simulink model "flightControlSystemV2"  (R2023a)
settings: Solver=ode3  StartTime=0  StopTime=TFinal  FixedStep=Ts  RelTol=1e-3  EnableMultiTasking=on
undefined symbols (not defined in the file or in its folder): codertarget, Controller, DiscIntNeverNeededParam, Discrete, Estimator, g, gray, init, orient_ref, pos_ref, Sensors, Time, Ts, var_acc_angle_N, var_bias_gyr_N, var_gyro_p_N, Vehicle
libraries: simulink x37, slpidlib x4, ctrlSharedLib x4, sharedtransform x3, parrotlib x1
(part 3 of 3)

== matlab function flightControlSystemV2/Image Processing System/MATLAB Function2 ==
  data: BW input; R input; G input; B input; state input; lineSteps input; len_center output; turn_angle output; state output; lineSteps output; R_out output; G_out output; B_out output; turn_angle input; turn input; turn output; correction output; angle input; angle output
function [len_center, turn_angle, state, lineSteps, R_out, G_out, B_out, turn, correction, angle] = droneGuidanceLines(BW, R, G, B, state, lineSteps, turn_angle, turn, angle)
    % Get image dimensions
    [rows, cols] = size(BW);

    turn_detected = false;
    turn_direction = 0;
    end_point_1 = [0,0];
    end_point_2 = [0,0];
    pinkColor = [255, 105, 180]; % RGB values for pink color
    greenColor = [0, 255, 0]; % RGB values for green color
    correction_thresh = 0.9;
    correction = 0;




    if state == 5
        turn = 0;
        state = 1;
    end
    
    % Define the drone's position (center of the image)
    drone_position = [round(rows/2), round(cols/2)];
    

    % Lengths of lines initialized to 0
    len_center = 0;
    len_left = 0;
    len_right = 0;
    len_left_or = 0;
    len_right_or = 0;
    len_back_left = 0;
    len_back_right = 0;
    len_left_corr = 0;
    len_right_corr = 0;
    
     % Step sizes for each line based on lineSteps array
    step_center = lineSteps(1,:);
    step_left = lineSteps(2,:);
    step_right = lineSteps(3,:);
    step_left_or = lineSteps(4,:);
    step_right_or = lineSteps(5,:);
    step_back_left = lineSteps(6,:);
    step_back_right = lineSteps(7,:);
    step_left_corr = [-step_center(2), step_center(1)]; 
    step_right_corr = [step_center(2), -step_center(1)]; 


    
    % Flags to check if lines should continue
    continue_center = true;
    continue_left = true;
    continue_right = true;
    continue_left_or = true;
    continue_right_or = true;
    continue_back_left = true;
    continue_back_right = true;
    continue_left_corr = true;
    continue_right_corr = true;



    % Initialize RGB values and lengths
    [len_center, R, G, B] = traceLine(drone_position, step_center, BW, R, G, B, pinkColor);
    [len_left, R, G, B] = traceLine(drone_position, step_left, BW, R, G, B, greenColor);
    [len_right, R, G, B] = traceLine(drone_position, step_right, BW, R, G, B, greenColor);
    [len_left_or, R, G, B] = traceLine(drone_position, step_left_or, BW, R, G, B, greenColor);
    [len_right_or, R, G, B] = traceLine(drone_position, step_right_or, BW, R, G, B, greenColor);
    [len_back_left, R, G, B] = traceLine(drone_position, step_back_left, BW, R, G, B, greenColor);
    [len_back_right, R, G, B] = traceLine(drone_position, step_back_right, BW, R, G, B, greenColor);

    % Compute the end point of the frontal line (center line)
    end_point_frontal = drone_position + (len_center * 0.9) * step_center;
    [len_left_corr, R, G, B] = traceLine(end_point_frontal, step_left_corr, BW, R, G, B, pinkColor);
    [len_right_corr, R, G, B] = traceLine(end_point_frontal, step_right_corr, BW, R, G, B, pinkColor);




    % Threshold percentage for significant difference
    threshold_percentage = 0.35;
    
    % Check for left turn
    if (len_left > (1 + threshold_percentage) * len_right) || (len_left_or > (1 + threshold_percentage) * len_right_or)
        end_point_1 = [];
        end_point_2 = [];
        turn_direction = 1;
        
        % New logic for determining type of left turn
        if len_center <= 30
            % Check for soft turn
            if len_back_left < 40 && len_left > len_center
                if len_left >= 60
                    end_point_2 = round(drone_position + len_center*step_center);
                    end_point_1 = round(drone_position + len_right*step_right);
                    turn = 1;  % soft turn
                    turn_detected = true;
                    % Color the center and right diagonal lines light blue
                    for i = 1:len_center
                        new_point = round(drone_position + i*step_center);
                        R(new_point(1), new_point(2)) = 173;
                        G(new_point(1), new_point(2)) = 216;
                        B(new_point(1), new_point(2)) = 230;
                    end
                    for i = 1:len_right
                        new_point = round(drone_position + i*step_right);
                        R(new_point(1), new_point(2)) = 173;
                        G(new_point(1), new_point(2)) = 216;
                        B(new_point(1), new_point(2)) = 230;
                    end
                else
                    end_point_1 = round(drone_position + len_center*step_center);
                    end_point_2 = round(drone_position + len_left*step_left);
                    turn_detected = true;
                    % Color the center and left diagonal lines light blue
                    for i = 1:len_center
                        new_point = round(drone_position + i*step_center);
                        R(new_point(1), new_point(2)) = 173;
                        G(new_point(1), new_point(2)) = 216;
                        B(new_point(1), new_point(2)) = 230;
                    end
                    for i = 1:len_left
                        new_point = round(drone_position + i*step_left);
                        R(new_point(1), new_point(2)) = 173;
                        G(new_point(1), new_point(2)) = 216;
                        B(new_point(1), new_point(2)) = 230;
                    end
                end
            else
                end_point_1 = round(drone_position + len_left*step_left);
                end_point_2 = round(drone_position + len_left_or*step_left_or);
                turn = 2;  % hard turn
                turn_detected = true;
                % Hard Turn: Color the left orthogonal and left diagonal lines orange
                for i = 1:len_left
                    new_point = round(drone_position + i*step_left);
                    R(new_point(1), new_point(2)) = 255;
                    G(new_point(1), new_point(2)) = 165;
                    B(new_point(1), new_point(2)) = 0;
                end
                for i = 1:len_left_or
                    new_point = round(drone_position + i*step_left_or);
                    R(new_point(1), new_point(2)) = 255;
                    G(new_point(1), new_point(2)) = 165;
                    B(new_point(1), new_point(2)) = 0;
                end
            end
        end
    % Check for right turn based on the previous logic
    elseif (len_right > (1 + threshold_percentage) * len_left) || (len_right_or > (1 + threshold_percentage) * len_left_or)
        % Logic for determining type of turn
        end_point_1 = [];
        end_point_2 = [];
        turn_direction = 2;
        if len_center <= 30
            % Check for soft turn
            if len_back_right < 40 && len_right > len_center
                if len_right >= 60
                    end_point_2 = round(drone_position + len_center*step_center);
                    end_point_1 = round(drone_position + len_left*step_left);
                    turn = 1;
                    turn_detected = true;
                    % Color the center and left diagonal lines light blue
                    for i = 1:len_center
                        new_point = round(drone_position + i*step_center);
                        R(new_point(1), new_point(2)) = 173;
                        G(new_point(1), new_point(2)) = 216;
                        B(new_point(1), new_point(2)) = 230;
                    end
                    for i = 1:len_left
                        new_point = round(drone_position + i*step_left);
                        R(new_point(1), new_point(2)) = 173;
                        G(new_point(1), new_point(2)) = 216;
                        B(new_point(1), new_point(2)) = 230;
                    end
                else
                    end_point_1 = round(drone_position + len_center*step_center);
                    end_point_2 = round(drone_position + len_right*step_right);
                    turn_detected = true;
                    % Color the center and right diagonal lines light blue
                    for i = 1:len_center
                        new_point = round(drone_position + i*step_center);
                        R(new_point(1), new_point(2)) = 173;
                        G(new_point(1), new_point(2)) = 216;
                        B(new_point(1), new_point(2)) = 230;
                    end
                    for i = 1:len_right
                        new_point = round(drone_position + i*step_right);
                        R(new_point(1), new_point(2)) = 173;
                        G(new_point(1), new_point(2)) = 216;
                        B(new_point(1), new_point(2)) = 230;
                    end
                end
            else
                end_point_1 = round(drone_position + len_right*step_right);
                end_point_2 = round(drone_position + len_right_or*step_right_or);
                turn = 2;
                turn_detected = true;
                % Hard Turn: Color the right orthogonal and right diagonal lines orange
                for i = 1:len_right
                    new_point = round(drone_position + i*step_right);
                    R(new_point(1), new_point(2)) = 255;
                    G(new_point(1), new_point(2)) = 165;
                    B(new_point(1), new_point(2)) = 0;
                end
                for i = 1:len_right_or
                    new_point = round(drone_position + i*step_right_or);
                    R(new_point(1), new_point(2)) = 255;
                    G(new_point(1), new_point(2)) = 165;
                    B(new_point(1), new_point(2)) = 0;
                end
            end
        end
    end
    
    if turn_detected && state == 1
        delta_y = end_point_2(2) - end_point_1(2);
        delta_x = end_point_2(1) - end_point_1(1);
        turn_angle = atan2(delta_y, delta_x);

        % Check if angle between the two end-points is zero (i.e., a 90-degree turn)
        if turn_angle == 0
            if turn_direction == 1 % Left turn
                turn_angle = -pi/2; % 90 degrees counter-clockwise
            elseif turn_direction == 2 % Right turn
                turn_angle = pi/2; % 90 degrees clockwise
            end
        end

        % if turn == 1
        %     turn_angle = turn_angle - pi/2;
        % elseif turn == 2
        %     turn_angle = turn_angle + pi/2 ;
        % end
        state = 2;
    end
    
    if state == 2
        R_matrix = [cos(-turn_angle) -sin(-turn_angle); sin(-turn_angle) cos(-turn_angle)];
        if len_center <= 15
            % Rotate all direction vectors
            rotated_step_center = (R_matrix * step_center').';
            rotated_step_left = (R_matrix * step_left').';
            rotated_step_right = (R_matrix * step_right').';
            rotated_step_left_or = (R_matrix * step_left_or').';
            rotated_step_right_or = (R_matrix * step_right_or').';
            rotated_step_back_left = (R_matrix * step_back_left').';
            rotated_step_back_right = (R_matrix * step_back_right').';

            % Storing the rotated steps back to lineSteps array
            lineSteps(1,:) = rotated_step_center;
            lineSteps(2,:) = rotated_step_left;
            lineSteps(3,:) = rotated_step_right;
            lineSteps(4,:) = rotated_step_left_or;
            lineSteps(5,:) = rotated_step_right_or;
            lineSteps(6,:) = rotated_step_back_left;
            lineSteps(7,:) = rotated_step_back_right;

            % Change state to turning so new angle is sent to path planning
            state = 3;
        end
    end
    
    % Correction State
    if state == 3
        corr_angle = 0.0174533;
        
        % Calculate differenc ein line lenght
        if len_left_corr > len_right_corr
            corr_dir = "left";
            len_diff = len_right_corr / len_left_corr;
        else
            corr_dir = "right";
            len_diff = len_left_corr / len_right_corr;
        end

        if len_diff <= correction_thresh
            if corr_dir == "left"
                turn_angle = turn_angle - corr_angle;
                correction = -corr_angle;
            elseif corr_dir == "right"
                turn_angle = turn_angle + corr_angle;
                correction = corr_angle;
            end

            % R2_matrix = [cos(-correction) -sin(-correction); sin(-correction) cos(-correction)];
            % 
            % % Rotate all direction vectors
            % rotated_step_center = (R2_matrix * step_center').';
            % rotated_step_left = (R2_matrix * step_left').';
            % rotated_step_right = (R2_matrix * step_right').';
            % rotated_step_left_or = (R2_matrix * step_left_or').';
            % rotated_step_right_or = (R2_matrix * step_right_or').';
            % rotated_step_back_left = (R2_matrix * step_back_left').';
            % rotated_step_back_right = (R2_matrix * step_back_right').';
            % 
            % % Storing the rotated steps back to lineSteps array
            % lineSteps(1,:) = rotated_step_center;
            % lineSteps(2,:) = rotated_step_left;
            % lineSteps(3,:) = rotated_step_right;
            % lineSteps(4,:) = rotated_step_left_or;
            % lineSteps(5,:) = rotated_step_right_or;
            % lineSteps(6,:) = rotated_step_back_left;
            % lineSteps(7,:) = rotated_step_back_right;
        else
            state = 4;
        end
    end

    % Split RGB channels for output
    R_out = R;
    G_out = G;
    B_out = B;
end


% Helper Functions
function colorLines(drone_position, len, step, R, G, B, color, turn_type)
    disp(['colorLines called for ', turn_type, ' turn']);
    [rows, cols] = size(R); % get image dimensions
    for i = 1:len
        new_point = round(drone_position + i*step);
        if new_point(1) > 0 && new_point(2) > 0 && new_point(1) <= rows && new_point(2) <= cols
            R(new_point(1), new_point(2)) = color(1);
            G(new_point(1), new_point(2)) = color(2);
            B(new_point(1), new_point(2)) = color(3);
        end
    end
end


function [len, R, G, B] = traceLine(drone_position, step, BW, R, G, B, lineColor)
    len = 0;
    [rows, cols] = size(BW);
    continue_trace = true;
    for i = 1:max(rows,cols)
        new_point = round(drone_position + i*step);
        if new_point(1) > 0 && new_point(2) > 0 && new_point(1) <= rows && new_point(2) <= cols && BW(new_point(1), new_point(2)) == 1
            R(new_point(1), new_point(2)) = lineColor(1);
            G(new_point(1), new_point(2)) = lineColor(2);
            B(new_point(1), new_point(2)) = lineColor(3);
            len = len + 1;
        else
            continue_trace = false;
        end
        
        if ~continue_trace
            break;
        end
    end
end


function [x, y] = ddaLine(x1, y1, x2, y2)
    dx = x2 - x1;
    dy = y2 - y1;
    
    step = max(abs(dx), abs(dy));
    
    x_inc = dx / step;
    y_inc = dy / step;
    
    x = x1;
    y = y1;
    
    result_x = [];
    result_y = [];
    
    for i = 0:step
        result_x = [result_x; round(x)];
        result_y = [result_y; round(y)];
        x = x + x_inc;
        y = y + y_inc;
    end
    
    x = result_x;
    y = result_y;
end

== matlab function flightControlSystemV2/Image Processing System/MATLAB Function ==
  data: I input; BW output
function BW = maskImg(I)

% Define thresholds for channel 1 based on histogram settings
channel1Min = 246.000;
channel1Max = 255.000;

% Define thresholds for channel 2 based on histogram settings
channel2Min = 0.000;
channel2Max = 232.000;

% Define thresholds for channel 3 based on histogram settings
channel3Min = 0.000;
channel3Max = 128.000;

% Create mask based on chosen histogram thresholds
sliderBW = (I(:,:,1) >= channel1Min ) & (I(:,:,1) <= channel1Max) & ...
    (I(:,:,2) >= channel2Min ) & (I(:,:,2) <= channel2Max) & ...
    (I(:,:,3) >= channel3Min ) & (I(:,:,3) <= channel3Max);
BW = sliderBW;

end

== matlab function flightControlSystemV2/Control System/Controller/Position Controller/Position error transformation (Earth to Body frame) ==
  data: yaw input; xy_err_earth input; xy_err_body output
function xy_err_body = fcn(yaw,xy_err_earth)

transformation = [cos(yaw), sin(yaw); -sin(yaw),  cos(yaw)];
xy_err_body = transformation * xy_err_earth;


end
